simulink model "ModelProd"  (Simulink 7.7)
settings: Solver=ode45  StartTime=0.0  StopTime=inf  RelTol=1e-3
libraries: vrlib x2, aerolibatmos2 x1, simulink x1, aerolibgravity2 x1
settings Model: Creator=Artem  LastModifiedBy=Artem

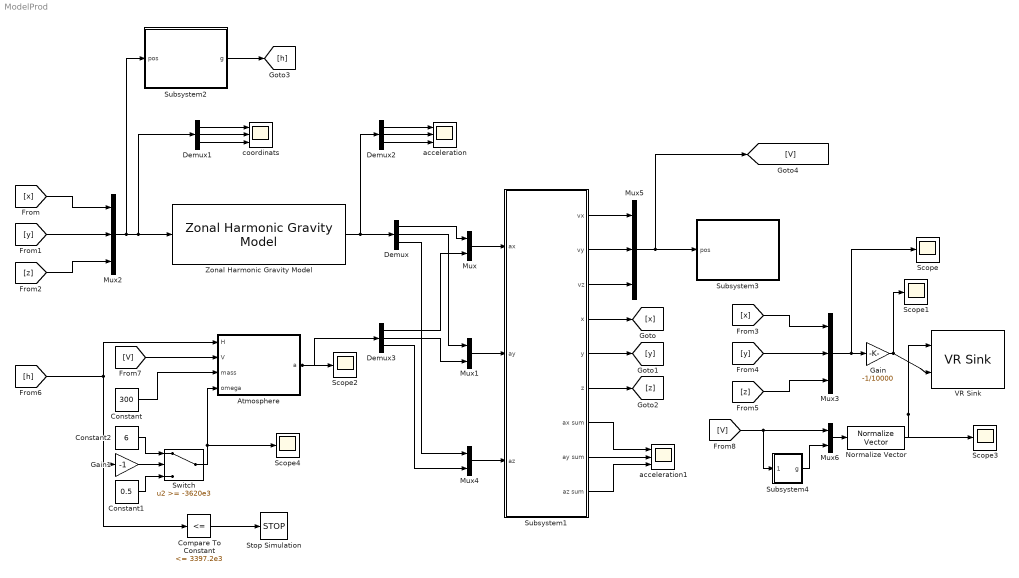
== system ModelProd ==
  Atmosphere : Subsystem
  Compare To Constant : simulink/Logic and Bit Operations/Compare To Constant  SystemSampleTime=-1  relop=<=  const=3397.2e3  LogicOutDataTypeMode=boolean
  Constant : Constant  Value=300
  Constant1 : Constant  Value=0.5
  Constant2 : Constant  Value=6
  Demux{,1..3} (4 alike) : Demux  Outputs=3
  Gain : Gain  Gain=-1/10000
  Gain1 : Gain  Gain=-1
  Mux{,1,4,6} (4 alike) : Mux  Inputs=2
  Mux2 : Mux  Inputs=3
  Mux3 : Mux  Inputs=3
  Mux5 : Mux  Inputs=3
  Normalize Vector : vrlib/Utilities/Normalize Vector  SystemSampleTime=-1  maxzero=0
  Scope{,1..4} (5 alike) : Scope
      Scope settings: SaveName=ScopeData2
      Scope1 settings: YMin=-50  YMax=600  SaveName=ScopeData4
      Scope2 settings: SaveName=ScopeData5
      Scope3 settings: SaveName=ScopeData6
      Scope4 settings: YMin=0.5  YMax=0.5  SaveName=ScopeData7
  Stop Simulation : Stop
  Subsystem1 : Subsystem
  Subsystem2 : Subsystem
  Subsystem3 : Subsystem
  Subsystem4 : Subsystem
  Switch : Switch  Threshold=-3620e3
  VR Sink : vrlib/VR Sink  SampleTime=0.1  ViewEnable=on  RemoteChange=off  RemoteView=on  FieldsWritten=Ship.rotation.4.1.1.double#Ship.translation.3.1.1.double  WorldFileName=vrplanets.wrl  WorldDescription=Planets  AutoView=off  VideoDimensions=[]
  Zonal Harmonic Gravity Model : aerolibgravity2/Zonal Harmonic Gravity Model  SystemSampleTime=-1  units=Metric (MKS)  degree=3  action=Warning  ptype=Mars  R=3397200  GM=43050000000000  jvalue=[1.9640000e-003 3.6000000e-005]
  acceleration : Scope  NumInputPorts=3
      settings: YMin=0~-5~-5  YMax=2.2e+021~5~5  SaveName=ScopeData3
  acceleration1 : Scope  NumInputPorts=3
      settings: YMin=0~-5~-5  YMax=2.2e+021~5~5  SaveName=ScopeData8
  coordinats : Scope  NumInputPorts=3
      settings: YMin=-347500~6.495e+006~44.525  YMax=-317500~6.5175e+006~44.875
  wires:
  Mux2/1 -> Subsystem2/1(pos), Demux1/1, Zonal Harmonic Gravity Model/1
  [y] -> Mux2/2
  [z] -> Mux2/3
  [x] -> Mux2/1
  Subsystem1/4(x) -> [x]
  Subsystem1/6(z) -> [z]
  Subsystem1/5(y) -> [y]
  [y] -> Mux3/2
  [z] -> Mux3/3
  [x] -> Mux3/1
  Mux3/1 -> Gain/1, Scope/1
  Zonal Harmonic Gravity Model/1 -> Demux2/1, Demux/1
  Demux1/1 -> coordinats/1
  Demux1/2 -> coordinats/2
  Demux1/3 -> coordinats/3
  Demux2/1 -> acceleration/1
  Demux2/2 -> acceleration/2
  Demux2/3 -> acceleration/3
  Subsystem1/1(vx) -> Mux5/1
  Mux/1 -> Subsystem1/1(ax)
  Mux4/1 -> Subsystem1/3(az)
  Mux1/1 -> Subsystem1/2(ay)
  Demux/1 -> Mux/1
  Demux/2 -> Mux1/1
  Demux/3 -> Mux4/1
  [h] -> Atmosphere/1(H), Compare To Constant/1, Gain1/1
  Compare To Constant/1 -> Stop Simulation/1
  Subsystem2/1(g) -> [h]
  Subsystem1/2(vy) -> Mux5/2
  Subsystem1/3(vz) -> Mux5/3
  Mux5/1 -> Subsystem3/1(pos), [V]
  Gain/1 -> Scope1/1, VR Sink/2
  [V] -> Atmosphere/2(V)
  Atmosphere/1(a) -> Scope2/1, Demux3/1
  Constant/1 -> Atmosphere/3(mass)
  Demux3/1 -> Mux/2
  Demux3/2 -> Mux1/2
  Demux3/3 -> Mux4/2
  Normalize Vector/1 -> VR Sink/1, Scope3/1
  [V] -> Mux6/1, Subsystem4/1(pos)
  Mux6/1 -> Normalize Vector/1
  Subsystem4/1(g) -> Mux6/2
  Switch/1 -> Atmosphere/4(omega), Scope4/1
  Constant1/1 -> Switch/3
  Constant2/1 -> Switch/1
  Gain1/1 -> Switch/2
  Subsystem1/7(ax sum) -> acceleration1/1
  Subsystem1/8(ay sum) -> acceleration1/2
  Subsystem1/9(az sum) -> acceleration1/3

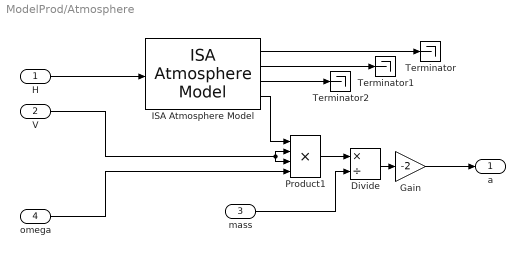
== system ModelProd/Atmosphere ==
  H : Inport
  V : Inport  Port=2
  mass : Inport  Port=3
  omega : Inport  Port=4
  Divide : Product  Inputs=*/
  Gain : Gain  Gain=-2
  ISA Atmosphere Model : aerolibatmos2/ISA Atmosphere Model  SystemSampleTime=-1  custom=on  g=3.72  gamma=2  R=188.92  L=0.0198  h_trop=25000  h_strat=50000  rho0=0.015  P0=800  T0=218
  Product1 : Product  Inputs=4  RndMeth=Zero
  Terminator : Terminator
  Terminator1 : Terminator
  Terminator2 : Terminator
  a : Outport
  wires:
  ISA Atmosphere Model/1 -> Terminator/1
  ISA Atmosphere Model/2 -> Terminator1/1
  ISA Atmosphere Model/3 -> Terminator2/1
  V/1 -> Product1/2, Product1/3
  omega/1 -> Product1/4
  Product1/1 -> Divide/1
  mass/1 -> Divide/2
  Divide/1 -> Gain/1
  Gain/1 -> a/1
  H/1 -> ISA Atmosphere Model/1
  ISA Atmosphere Model/4 -> Product1/1

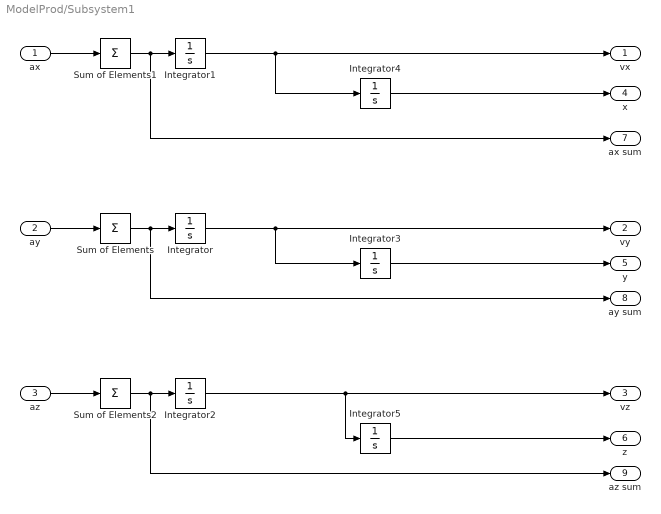
== system ModelProd/Subsystem1 ==
  ax : Inport
  ay : Inport  Port=2
  az : Inport  Port=3
  Integrator : Integrator  InitialCondition=4200
  Integrator1 : Integrator  InitialCondition=1360
  Integrator2 : Integrator
  Integrator3 : Integrator  InitialCondition=-3660e3
  Integrator4 : Integrator  InitialCondition=-3660e3
  Integrator5 : Integrator
  Sum of Elements : Sum  Inputs=+
  Sum of Elements1 : Sum  Inputs=+
  Sum of Elements2 : Sum  Inputs=+
  vx : Outport
  vy : Outport  Port=2
  vz : Outport  Port=3
  x : Outport  Port=4
  y : Outport  Port=5
  z : Outport  Port=6
  ax sum : Outport  Port=7
  ay sum : Outport  Port=8
  az sum : Outport  Port=9
  wires:
  ay/1 -> Sum of Elements/1
  ax/1 -> Sum of Elements1/1
  Sum of Elements1/1 -> Integrator1/1, ax sum/1
  az/1 -> Sum of Elements2/1
  Sum of Elements2/1 -> Integrator2/1, az sum/1
  Sum of Elements/1 -> Integrator/1, ay sum/1
  Integrator2/1 -> vz/1, Integrator5/1
  Integrator5/1 -> z/1
  Integrator3/1 -> y/1
  Integrator/1 -> Integrator3/1, vy/1
  Integrator4/1 -> x/1
  Integrator1/1 -> Integrator4/1, vx/1

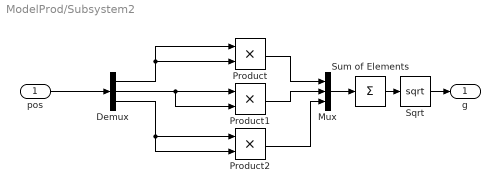
== system ModelProd/Subsystem2 ==
  pos : Inport
  Demux : Demux  Outputs=3
  Mux : Mux  Inputs=3
  Product : Product  RndMeth=Zero
  Product1 : Product  RndMeth=Zero
  Product2 : Product  RndMeth=Zero
  Sqrt : Sqrt  SaturateOnIntegerOverflow=on
  Sum of Elements : Sum  Inputs=+
  g : Outport
  wires:
  pos/1 -> Demux/1
  Demux/1 -> Product/1, Product/2
  Demux/2 -> Product1/1, Product1/2
  Demux/3 -> Product2/1, Product2/2
  Product/1 -> Mux/1
  Product1/1 -> Mux/2
  Product2/1 -> Mux/3
  Mux/1 -> Sum of Elements/1
  Sum of Elements/1 -> Sqrt/1
  Sqrt/1 -> g/1

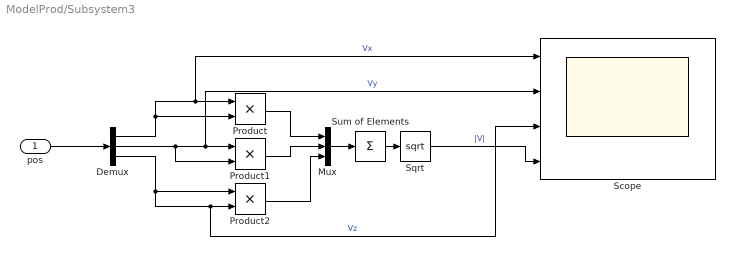
== system ModelProd/Subsystem3 ==
  pos : Inport
  Demux : Demux  Outputs=3
  Mux : Mux  Inputs=3
  Product : Product  RndMeth=Zero
  Product1 : Product  RndMeth=Zero
  Product2 : Product  RndMeth=Zero
  Scope : Scope  NumInputPorts=4
      settings: YMin=272.88~271.257~0.017125~384.765  YMax=272.955~271.263~0.017525~384.825
  Sqrt : Sqrt  SaturateOnIntegerOverflow=on
  Sum of Elements : Sum  Inputs=+
  wires:
  pos/1 -> Demux/1
  Demux/1 -> Product/2, Product/1, Scope/1  "Vx"
  Demux/2 -> Product1/2, Product1/1, Scope/2  "Vy"
  Demux/3 -> Product2/1, Product2/2, Scope/3  "Vz"
  Product/1 -> Mux/1
  Product1/1 -> Mux/2
  Product2/1 -> Mux/3
  Mux/1 -> Sum of Elements/1
  Sum of Elements/1 -> Sqrt/1
  Sqrt/1 -> Scope/4  "|V|"

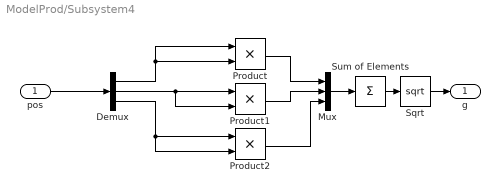
== system ModelProd/Subsystem4 ==
  pos : Inport
  Demux : Demux  Outputs=3
  Mux : Mux  Inputs=3
  Product : Product  RndMeth=Zero
  Product1 : Product  RndMeth=Zero
  Product2 : Product  RndMeth=Zero
  Sqrt : Sqrt  SaturateOnIntegerOverflow=on
  Sum of Elements : Sum  Inputs=+
  g : Outport
  wires:
  Sqrt/1 -> g/1
  Sum of Elements/1 -> Sqrt/1
  Mux/1 -> Sum of Elements/1
  Product2/1 -> Mux/3
  Product1/1 -> Mux/2
  Product/1 -> Mux/1
  Demux/3 -> Product2/2, Product2/1
  Demux/2 -> Product1/2, Product1/1
  Demux/1 -> Product/2, Product/1
  pos/1 -> Demux/1
